simulink model "Segway"  (R2019a)
settings: Solver=FixedStepAuto  StartTime=0.0  StopTime=30  FixedStep=0.001  RelTol=1e-3
values from neighbouring files (symbols this model uses):
  A = [0              1   0   0 ... (first row only)    [Legway_main.m]
  B = [0  0 ... (first row only)    [Legway_main.m]
  B_T0 = [0 ... (first row only)    [Legway_main.m]
  F = 0    [Legway_main.m]
  g = 9.81    [Legway_main.m]
  K = acker(A,B_T0, des_poles)    [Legway_main.m]
  K_speed = place(A,B_T0, des_poles2)    [Legway_main.m]
  l = 1    [Legway_main.m]
  M = 1    [Legway_main.m]
  m = 1    [Legway_main.m]
  T = 0    [Legway_main.m]
  X0 = [pi;0;0;0]    [Legway_main.m]
  X_des = [0;0;10;0]    [Legway_main.m]
  X_speed = [0;0;0;1]    [Legway_main.m]
settings Model: Creator=boiti  LastModifiedBy=boiti

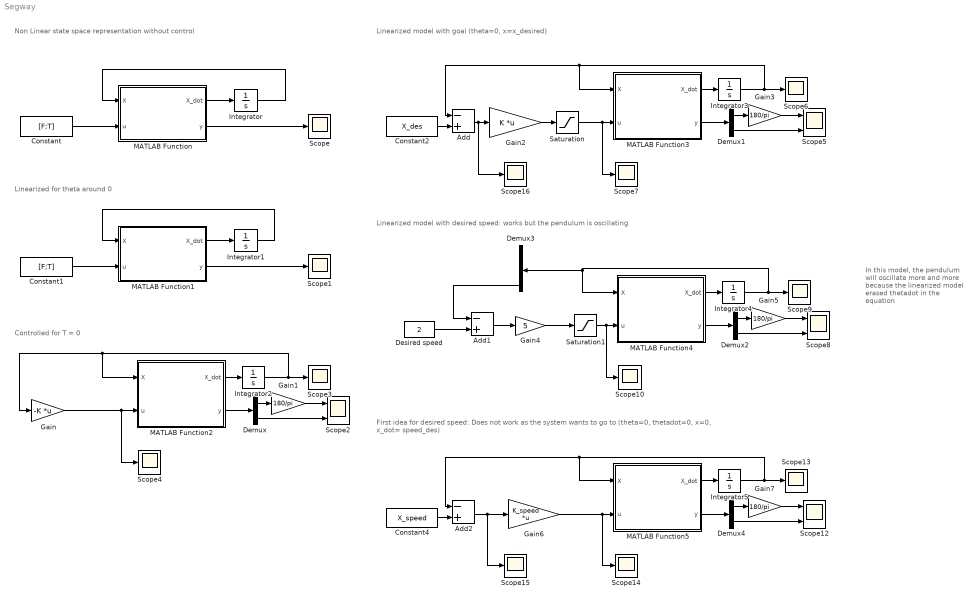
== system Segway ==
  note: In this model, the pendulum will oscillate more and more because the linearized model erased thetadot in the equation
  note: Linearized model with goal (theta=0, x=x_desired)
  note: Linearized for theta around 0
  note: Non Linear state space representation without control
  note: Controlled for T = 0
  note: Linearized model with desired speed: works but the pendulum is oscillating
  note: First idea for desired speed: Does not work as the system wants to go to (theta=0, thetadot=0, x=0, x_dot= speed_des)
  Add : Sum  Inputs=-+
  Add1 : Sum  Inputs=-+
  Add2 : Sum  Inputs=-+
  Constant : Constant  Value=[F;T]
  Constant1 : Constant  Value=[F;T]
  Constant2 : Constant  Value=X_des
  Constant4 : Constant  Value=X_speed
  Demux{,1..2,4} (4 alike) : Demux  Outputs=2
  Demux3 : Demux
  Desired speed : Constant  Value=2
  Gain : Gain  Gain=-K  Multiplication=Matrix(K*u)
  Gain{1,3,5,7} (4 alike) : Gain  Gain=180/pi
  Gain2 : Gain  Gain=K  Multiplication=Matrix(K*u)
  Gain4 : Gain  Gain=5
  Gain6 : Gain  Gain=K_speed  Multiplication=Matrix(K*u)
  Integrator : Integrator  InitialCondition=X0  WrapState=on  WrappedStateUpperValue=[2*pi;inf;inf;inf]  WrappedStateLowerValue=[0;-inf;-inf;-inf]
  Integrator1 : Integrator  InitialCondition=X0  WrapState=on  WrappedStateUpperValue=[2*pi;inf;inf;inf]  WrappedStateLowerValue=[0;-inf;-inf;-inf]
  Integrator{2..5} (4 alike) : Integrator  InitialCondition=X0  WrapState=on  WrappedStateUpperValue=[2*pi;inf;inf;inf]  WrappedStateLowerValue=[-2*pi;-inf;-inf;-inf]
  MATLAB Function : MATLAB Function  TreatAsAtomicUnit=on
  MATLAB Function1 : MATLAB Function  TreatAsAtomicUnit=on
  MATLAB Function2 : MATLAB Function  TreatAsAtomicUnit=on
  MATLAB Function3 : MATLAB Function  TreatAsAtomicUnit=on
  MATLAB Function4 : MATLAB Function  TreatAsAtomicUnit=on
  MATLAB Function5 : MATLAB Function  TreatAsAtomicUnit=on
  Saturation : Saturate  UpperLimit=50  LowerLimit=-50
  Saturation1 : Saturate  UpperLimit=50  LowerLimit=-50
  Scope{,1,3..4,6..7,9..10,13..16} (12 alike) : Scope
  Scope{2,5,8,12} (4 alike) : Scope  NumInputPorts=2
  wires:
  MATLAB Function/1(X_dot) -> Integrator/1
  Integrator/1 -> MATLAB Function/1(X)
  MATLAB Function/2(y) -> Scope/1
  Constant/1 -> MATLAB Function/2(u)
  MATLAB Function1/1(X_dot) -> Integrator1/1
  Integrator1/1 -> MATLAB Function1/1(X)
  MATLAB Function1/2(y) -> Scope1/1
  Constant1/1 -> MATLAB Function1/2(u)
  MATLAB Function2/1(X_dot) -> Integrator2/1
  Integrator2/1 -> Scope3/1, MATLAB Function2/1(X), Gain/1
  Gain/1 -> Scope4/1, MATLAB Function2/2(u)
  MATLAB Function2/2(y) -> Demux/1
  Demux/2 -> Scope2/2
  Demux/1 -> Gain1/1
  Gain1/1 -> Scope2/1
  Integrator3/1 -> Scope6/1, Add/1, MATLAB Function3/1(X)
  MATLAB Function3/1(X_dot) -> Integrator3/1
  Demux1/1 -> Gain3/1
  MATLAB Function3/2(y) -> Demux1/1
  Gain3/1 -> Scope5/1
  Demux1/2 -> Scope5/2
  Add/1 -> Scope16/1, Gain2/1
  Constant2/1 -> Add/2
  Gain2/1 -> Saturation/1
  Saturation/1 -> Scope7/1, MATLAB Function3/2(u)
  Gain5/1 -> Scope8/1
  MATLAB Function4/1(X_dot) -> Integrator4/1
  Integrator4/1 -> Scope9/1, MATLAB Function4/1(X), Demux3/1
  Demux2/2 -> Scope8/2
  MATLAB Function4/2(y) -> Demux2/1
  Add1/1 -> Gain4/1
  Desired speed/1 -> Add1/2
  Demux2/1 -> Gain5/1
  Saturation1/1 -> Scope10/1, MATLAB Function4/2(u)
  MATLAB Function5/1(X_dot) -> Integrator5/1
  Integrator5/1 -> Scope13/1, Add2/1, MATLAB Function5/1(X)
  Demux4/2 -> Scope12/2
  MATLAB Function5/2(y) -> Demux4/1
  Add2/1 -> Scope15/1, Gain6/1
  Gain7/1 -> Scope12/1
  Demux4/1 -> Gain7/1
  Constant4/1 -> Add2/2
  Gain6/1 -> Scope14/1, MATLAB Function5/2(u)
  Gain4/1 -> Saturation1/1
  Demux3/4 -> Add1/1

== matlab function Segway/MATLAB Function1 ==
  data: X input; X_dot output; u input; y output; A parameter; B parameter
function [X_dot, y] = Linear(X, u, A, B)
X_dot = A*X + B*u;
y = [X(1);X(3)];

== matlab function Segway/MATLAB Function ==
  data: X input; X_dot output; u input; y output; m parameter; M parameter; g parameter; l parameter
function [X_dot, y] = Non_Linear(X, u, m, M, g, l)
% X = [theta theta_dot x x_dot], u = [F T]
X_dot = [X(2);
    ((M+m)*g*l*sin(X(1)) - m*(l^2)*(X(2)^2)*cos(X(1))*sin(X(1)) + (M+m)*u(2)/m + l*cos(X(1))*u(1))*1/((M+m-(m*cos(X(1))^2))*l^2);
    X(4);
    (-m*l*(X(2)^2)*sin(X(1))+ m*g*cos(X(1))*sin(X(1)) + u(2)*cos(X(1))/l + u(1))*1/(M+m-(m*cos(X(1))^2))];

y = [X(1); X(3)];

== matlab function Segway/MATLAB Function2 ==
  data: X input; X_dot output; u input; y output; A parameter; B_T0 parameter
function [X_dot, y] = Linear_T0(X, u, A, B_T0)
X_dot = A*X + B_T0*u;
y = [X(1);X(3)];

== matlab function Segway/MATLAB Function3 ==
  data: X input; X_dot output; u input; y output; A parameter; B_T0 parameter
function [X_dot, y] = Linear_T0(X, u, A, B_T0)
X_dot = A*X + B_T0*u;
y = [X(1);X(3)];

== matlab function Segway/MATLAB Function4 ==
  data: X input; X_dot output; u input; y output; A parameter; B_T0 parameter
function [X_dot, y] = Linear_T0(X, u, A, B_T0)
X_dot = A*X + B_T0*u;
y = [X(1);X(3)];

== matlab function Segway/MATLAB Function5 ==
  data: X input; X_dot output; u input; y output; A parameter; B_T0 parameter
function [X_dot, y] = Linear_with_T(X, u, A, B_T0)
X_dot = A*X + B_T0*u;
y = [X(1);X(3)];
